simulink model "test1"  (Simulink 9.0)
settings: Solver=VariableStepAuto  StartTime=0.0  StopTime=10.0  RelTol=1e-3
settings Model: SuppressorTable=22 serialization::archive 11 0 6 0 0 0 11 0  Creator=flosch  LastModifiedBy=flosch
settings DataIOCC: SaveFormat=Dataset
settings OptimizationCC: LifeSpan=auto
settings DebuggingCC: UnderspecifiedInitializationDetection=Simplified  MergeDetectMultiDrivingBlocksExec=error  SFUnexpectedBacktrackingDiag=error  SFNoUnconditionalDefaultTransitionDiag=error  SFExecutionAtInitializationDiag=warning
settings HardwareCC: ProdBitPerPointer=64  ProdBitPerSizeT=64  ProdBitPerPtrDiffT=64  ProdLargestAtomicFloat=Float  ProdIntDivRoundTo=Zero  ProdEndianess=LittleEndian  ProdWordSize=64  ProdHWDeviceType=Intel->x86-64 (Windows64)
settings ModelReferenceCC: PropagateSignalLabelsOutOfModel=on
settings CodeAppCC: StateflowObjectComments=off
settings GRTTargetCC: TargetLangStandard=C99 (ISO)
settings ConfigComp: CovMetricSettings=dwe  CovHtmlReporting=off  CovSaveCumulativeToWorkspaceVar=off  CovSaveSingleToWorkspaceVar=off  CovExternalEMLEnable=on

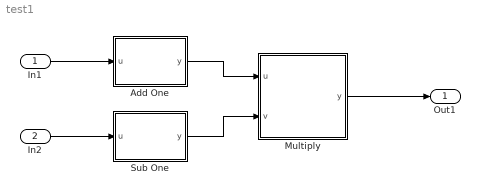
== system test1 ==
  In1 : Inport
  In2 : Inport  Port=2
  Add One : MATLAB Function  TreatAsAtomicUnit=on
  Multiply : MATLAB Function  TreatAsAtomicUnit=on
  Sub One : MATLAB Function  TreatAsAtomicUnit=on
  Out1 : Outport
  wires:
  Add One/1(y) -> Multiply/1(u)
  Sub One/1(y) -> Multiply/2(v)
  In1/1 -> Add One/1(u)
  In2/1 -> Sub One/1(u)
  Multiply/1(y) -> Out1/1

== matlab function Sub One ==
  data: u input double; y output double
function y = sub_one(u)

y = u - 1;

== matlab function Add One ==
  data: u input double; y output double
function y = add_one(u)

y = u + 1;

== matlab function Multiply ==
  data: u input double; y output double; v input double
function y = my_multiply(u, v)

y = u * v;
